simulink model "Modello_carroponte_validazione"  (R2024a)
settings: Solver=VariableStepAuto  StartTime=tempo(1)  StopTime=tempo(end)  FixedStep=dt  RelTol=1e-3
undefined symbols (not defined in the file): A, alpha_0, alpha_0_eq, alpha_dot_0, B, C, cc, cm, D, dinamica_alpha, g, L, mc, mm, xc_0, xc_0_eq, xc_dot_0
settings Model: Creator=smila  LastModifiedBy=smila

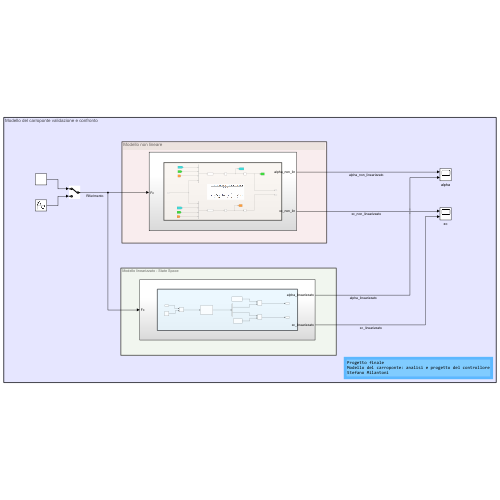
[thumbnail: Simulink's stored preview of the top-level diagram]
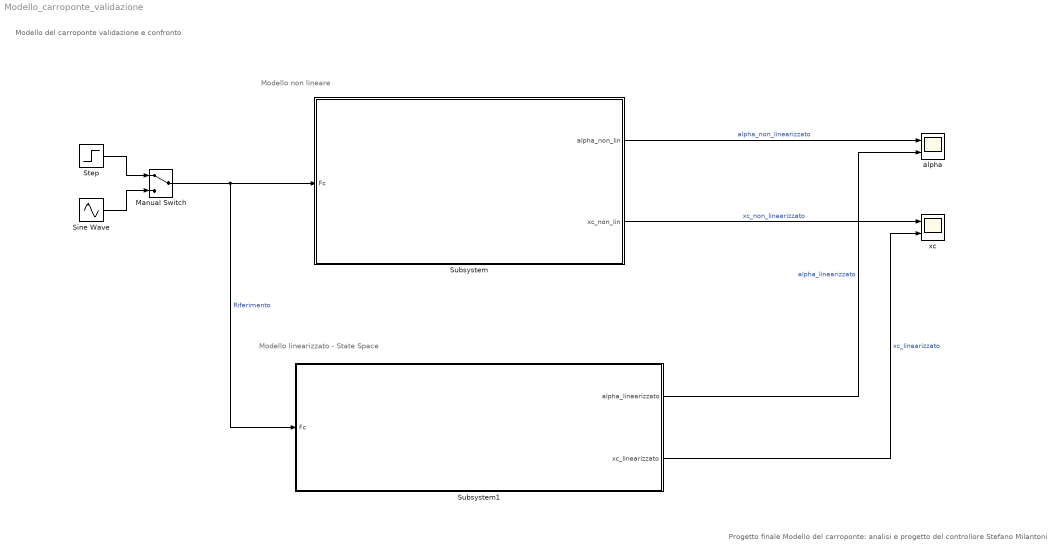
== system Modello_carroponte_validazione ==
  note: Modello del carroponte validazione e confronto
  note: Modello linearizzato - State Space
  note: Modello non lineare
  note: Progetto finale
      | Modello del carroponte: analisi e progetto del controllore
      | Stefano Milantoni
  Manual Switch : ManualSwitch
  Sine Wave : Sin  Amplitude=1e3  Frequency=2  SampleTime=0
  Step : Step  Time=15  SampleTime=0
  Subsystem : Subsystem
  Subsystem1 : Subsystem
  alpha : Scope  NumInputPorts=2
  xc : Scope  NumInputPorts=2
  wires:
  Subsystem/1(alpha_non_lin) -> alpha/1  "alpha_non_linearizzato"
  Subsystem/2(xc_non_lin) -> xc/1  "xc_non_linearizzato"
  Subsystem1/1(alpha_linearizzato) -> alpha/2  "alpha_linearizzato"
  Subsystem1/2(xc_linearizzato) -> xc/2  "xc_linearizzato"
  Step/1 -> Manual Switch/1
  Sine Wave/1 -> Manual Switch/2
  Manual Switch/1 -> Subsystem1/1(Fc), Subsystem/1(Fc)  "Riferimento"

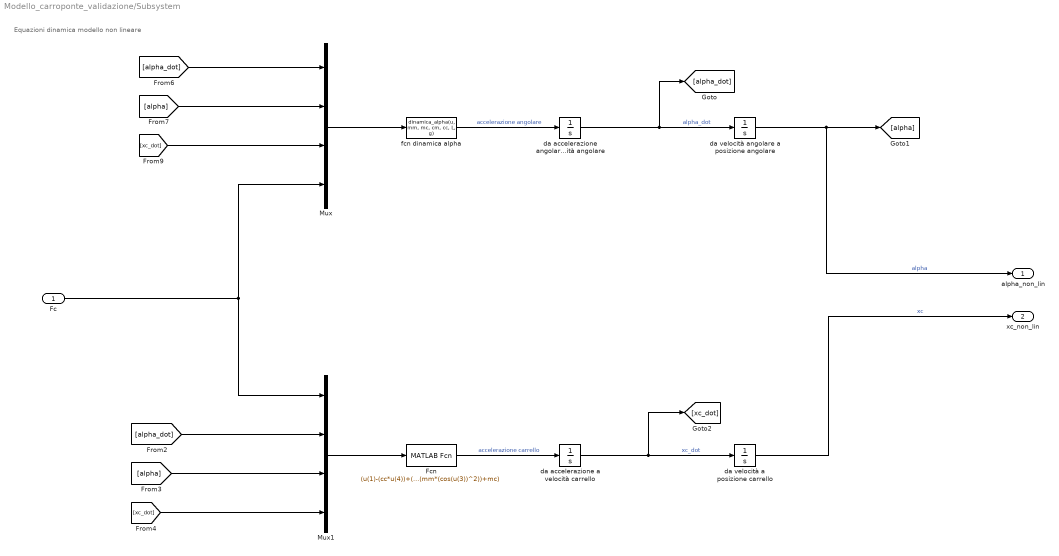
== system Modello_carroponte_validazione/Subsystem ==
  note: Equazioni dinamica modello non lineare
  Fc : Inport
  Fcn : MATLABFcn  MATLABFcn=(u(1)-(cc*u(4))+(mm*g*sin(u(3))*cos(u(3)))-(cm*u(4)*(cos(u(3))^2))+(mm*L*cos(u(3))*(u(2)^2)))/((mm*(cos(u(3))^2))+mc)
  Mux : Mux
  Mux1 : Mux
  da accelerazione a velocità carrello : Integrator  InitialCondition=xc_dot_0
  da accelerazione angolare a velocità angolare : Integrator  InitialCondition=alpha_dot_0
  da velocità a posizione carrello : Integrator  InitialCondition=xc_0
  da velocità angolare a posizione angolare : Integrator  InitialCondition=alpha_0
  fcn dinamica alpha : MATLABFcn  MATLABFcn=dinamica_alpha(u, mm, mc, cm, cc, L, g)
  alpha_non_lin : Outport
  xc_non_lin : Outport  Port=2
  wires:
  da accelerazione angolare a velocità angolare/1 -> da velocità angolare a posizione angolare/1, [alpha_dot]  "alpha_dot"
  da velocità angolare a posizione angolare/1 -> alpha_non_lin/1, [alpha]  "alpha"
  Mux1/1 -> Fcn/1
  [xc_dot] -> Mux1/4
  [alpha_dot] -> Mux1/2
  Mux/1 -> fcn dinamica alpha/1
  Fc/1 -> Mux1/1, Mux/4
  Fcn/1 -> da accelerazione a velocità carrello/1  "accelerazione carrello"
  da velocità a posizione carrello/1 -> xc_non_lin/1  "xc"
  da accelerazione a velocità carrello/1 -> da velocità a posizione carrello/1, [xc_dot]  "xc_dot"
  [alpha] -> Mux/2
  [alpha] -> Mux1/3
  [alpha_dot] -> Mux/1
  [xc_dot] -> Mux/3
  fcn dinamica alpha/1 -> da accelerazione angolare a velocità angolare/1  "accelerazione angolare"

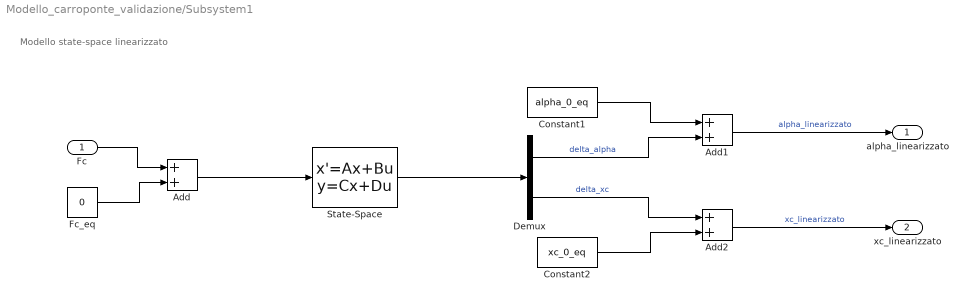
== system Modello_carroponte_validazione/Subsystem1 ==
  note: Modello state-space linearizzato
  Fc : Inport
  Add : Sum
  Add1 : Sum
  Add2 : Sum
  Constant1 : Constant  Value=alpha_0_eq
  Constant2 : Constant  Value=xc_0_eq
  Demux : Demux  Outputs=2
  Fc_eq : Constant  Value=0
  State-Space : StateSpace  A=A  B=B  C=C  D=D  InitialCondition=0
  alpha_linearizzato : Outport
  xc_linearizzato : Outport  Port=2
  wires:
  Constant1/1 -> Add1/1
  Add2/1 -> xc_linearizzato/1  "xc_linearizzato"
  Add/1 -> State-Space/1
  Fc_eq/1 -> Add/2
  State-Space/1 -> Demux/1
  Demux/2 -> Add2/1  "delta_xc"
  Constant2/1 -> Add2/2
  Demux/1 -> Add1/2  "delta_alpha"
  Add1/1 -> alpha_linearizzato/1  "alpha_linearizzato"
  Fc/1 -> Add/1
